simulink model "Control_discreto_Dom_tiempo"  (R2023b)
settings: Solver=VariableStepAuto  StartTime=0.0  StopTime=15  FixedStep=0.0001  MaxStep=1e-3  RelTol=1e-3
values from neighbouring files (symbols this model uses):
  ba = Jeq * n * wn    [PolosPID.m]
  id_consigna = 0.5    [RdLazoCorriente.m]
  ketita = double(sol.ketita_s)    [PIDPolosObsReducidoEst.m]    (also in PolosObsReducidoEst.m)
  kew = double(sol.kew_s)    [PIDPolosObsReducidoEst.m]    (also in PolosObsReducidoEst.m)
  kewint = double(sol.kewint_s)    [PIDPolosObsReducidoEst.m]    (also in PolosObsReducidoEst.m = 0)
  Ksa = Jeq * n * wn^2    [PolosPID.m]
  Ksia = Jeq * wn^3    [PolosPID.m]
  Ra_prima = Lq/Tau    [RaLazoControlCorriente.m]
  Rd_prima = Ld/Tau_d    [RdLazoCorriente.m]
  Ts = 0.0001    [TustinPID.m]
undefined symbols (not defined in the file or in its folder): alfa, beq, Cts, ee_sli_rtmsupport, g, gcbh, i0_consigna, id0, io0, iq0, Ismax, Isnom, Jeq, KEeq, kl, KTeq, lambda_m, Ld, Lls, Lq, Pp, r, R0_prima, Rs, Rts_amb, tita0, Tqnom, Ts0, Tsmax, Vflnom, Wlnom, wm0, Wmnom
libraries: SignalEditorBlockLib x3, dspsigops x1, spsabctoAlphaBetaZeroLib x1
settings Model: Creator=Julian  LastModifiedBy=Gustavo

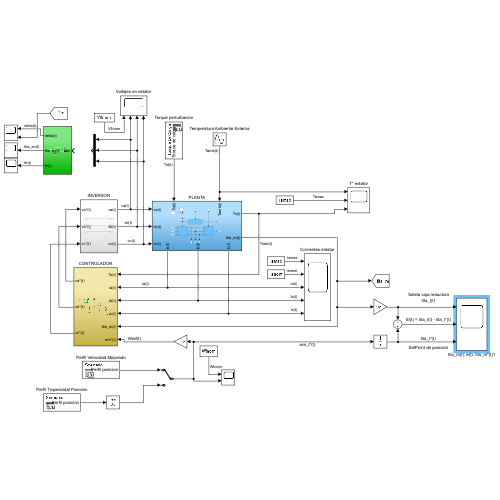
[thumbnail: Simulink's stored preview of the top-level diagram]
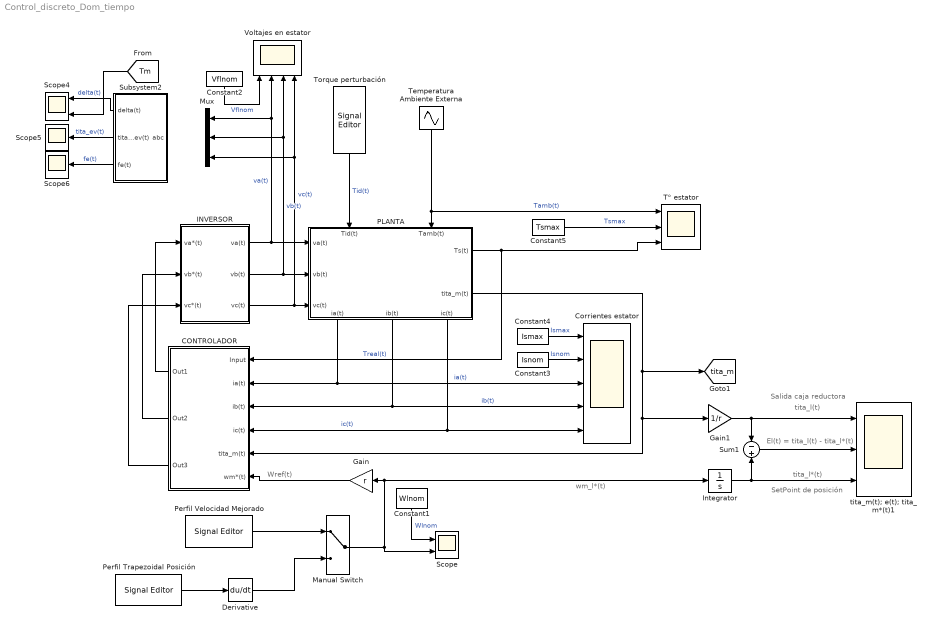
== system Control_discreto_Dom_tiempo ==
  note: SetPoint de posición
  note: Wref(t)
  note: Salida caja reductora
  note: El(t) = tita_l(t) - tita_l*(t)
  note: tita_l*(t)
  note: wm_l*(t)
  note: tita_l(t)
  CONTROLADOR : Subsystem
  Constant1 : Constant  Value=Wlnom
  Constant2 : Constant  Value=Vflnom
  Constant3 : Constant  Value=Isnom
  Constant4 : Constant  Value=Ismax
  Constant5 : Constant  Value=Tsmax
  Corrientes estator : Scope  NumInputPorts=5
  Derivative : Derivative
  Gain : Gain  Gain=r
  Gain1 : Gain  Gain=1/r
  INVERSOR : Subsystem
  Integrator : Integrator
  Manual Switch : ManualSwitch
  Mux : Mux  Inputs=3
  PLANTA : Subsystem
      settings: PortSchema="{\"entries\":[{\"content\":{\"sides\":[{\"content\":{\"connectorIds\":[\"In1\",\"In2\",\"In3\"]},\"type\":\"ConnectorPlacement.EquallySpacedRectSide\",\"uuid\":\"c9ff8e03-575d-49b6-9d53-263c6173ec7a\"},{\"content\":{\"connectorIds\":[\"Out1\",\"Out2\"],\"side\":\"RIGHT\"},\"type\":\"ConnectorPlacement.EquallySpacedRectSide\",\"uuid\":\"b812656a-111e-4032-91bd-eba1e3276cdf\"},{\"content\":{\"connectorIds\":[\"In4\",\"In5\"],\"side\":\"TOP\"},\"type\":\"ConnectorPlacement.EquallySpacedRectSide\",\"uuid\":\"1a03caaa-7f6e-4ad3-ab54-ee47607f786a\"},{\"content\":{\"connectorIds\":[\"Out3\",\"Out4\",\"Out5\"],\"side\":\"BOTTOM\"},\"type\":\"ConnectorPlacement.EquallySpacedRectSide\",\"uuid\":\"9d23a867-d392-4f38-a76b-2655c4618fc4\"}]},\"type\":\"ConnectorPlacement.EquallySpacedConnector\",\"uuid\":\"9323b1ce-1fa4-461e-b8aa-3e94b35b1dab\"}],\"packageUris\":[\"http://schema.mathworks.com/mf0/Connector/R2020b\"],\"version\":\"1.0\"}"
  Perfil Trapezoidal Posición : SignalEditorBlockLib/Signal Editor  FileName=Perfil trapezoidal de posicion.mat  ActiveScenario=Scenario  ActiveSignal=Perfil posicion  IsBus=off  OutputBusObjectStr=Bus: BusObject  SampleTime=0  ZeroCross=off  OutputAfterFinalValue=Setting to zero  Unit=inherit  PreserveSignalName=on  ApplySigPropsToAllScenarios=on  ApplySigPropsToAllSignals=off
  Perfil Velocidad Mejorado : SignalEditorBlockLib/Signal Editor  FileName=PerfilTrapezoidalVelocidadMejorado.mat  ActiveScenario=Scenario  ActiveSignal=Perfil posicion  IsBus=off  OutputBusObjectStr=Bus: BusObject  SampleTime=0  ZeroCross=off  OutputAfterFinalValue=Setting to zero  Unit=inherit  PreserveSignalName=on  ApplySigPropsToAllScenarios=on  ApplySigPropsToAllSignals=off
  Scope : Scope  NumInputPorts=2
  Scope4 : Scope  NumInputPorts=2
  Scope5 : Scope
  Scope6 : Scope
  Subsystem2 : Subsystem
  Sum1 : Sum  Inputs=-|+
  Temperatura Ambiente Externa : Sin  Bias=40  Frequency=2*pi/15  Phase=pi/2  SampleTime=0
  Torque perturbación : SignalEditorBlockLib/Signal Editor  FileName=Torque de carga Tdl(t).mat  ActiveScenario=TorqueDeCarga  ActiveSignal=Torque de carga  IsBus=off  OutputBusObjectStr=Bus: BusObject  SampleTime=0  ZeroCross=off  OutputAfterFinalValue=Setting to zero  Unit=N*m  PreserveSignalName=on  ApplySigPropsToAllScenarios=on  ApplySigPropsToAllSignals=off
  T° estator : Scope  NumInputPorts=3
  Voltajes en estator : Scope  NumInputPorts=4
  tita_m(t); e(t); tita_m*(t)1 : Scope  NumInputPorts=3
  tag scope: tita_m=global
  wires:
  INVERSOR/1(va(t)) -> PLANTA/1(va(t)), Voltajes en estator/2, Mux/1  "va(t)"
  INVERSOR/2(vb(t)) -> PLANTA/2(vb(t)), Mux/2, Voltajes en estator/3  "vb(t)"
  INVERSOR/3(vc(t)) -> Voltajes en estator/4, Mux/3, PLANTA/3(vc(t))  "vc(t)"
  CONTROLADOR/1(Out1) -> INVERSOR/1(va*(t))
  CONTROLADOR/2(Out2) -> INVERSOR/2(vb*(t))
  CONTROLADOR/3(Out3) -> INVERSOR/3(vc*(t))
  Gain/1 -> CONTROLADOR/6(wm*(t))
  PLANTA/2(tita_m(t)) -> CONTROLADOR/5(tita_m(t)), Gain1/1, [tita_m]
  Gain1/1 -> tita_m(t); e(t); tita_m*(t)1/1, Sum1/1
  Sum1/1 -> tita_m(t); e(t); tita_m*(t)1/2
  Integrator/1 -> Sum1/2, tita_m(t); e(t); tita_m*(t)1/3
  Temperatura Ambiente Externa/1 -> PLANTA/5(Tamb(t)), T° estator/1  "Tamb(t)"
  Torque perturbación/1 -> PLANTA/4(Tid(t))  "Tid(t)"
  PLANTA/5(ic(t)) -> Corrientes estator/5, CONTROLADOR/4(ic(t))  "ic(t)"
  PLANTA/4(ib(t)) -> Corrientes estator/4, CONTROLADOR/3(ib(t))  "ib(t)"
  PLANTA/3(ia(t)) -> Corrientes estator/3, CONTROLADOR/2(ia(t))  "ia(t)"
  Manual Switch/1 -> Integrator/1, Gain/1, Scope/2
  Perfil Trapezoidal Posición/1 -> Derivative/1
  Perfil Velocidad Mejorado/1 -> Manual Switch/1
  Constant1/1 -> Scope/1  "Wlnom"
  Constant2/1 -> Voltajes en estator/1  "Vflnom"
  Constant3/1 -> Corrientes estator/2  "Isnom"
  Constant4/1 -> Corrientes estator/1  "Ismax"
  Constant5/1 -> T° estator/2  "Tsmax"
  Derivative/1 -> Manual Switch/2
  PLANTA/1(Ts(t)) -> CONTROLADOR/1(Input), T° estator/3  "Treal(t)"
  Subsystem2/1(delta(t)) -> Scope4/1  "delta(t)"
  Subsystem2/2(tita_ev(t)) -> Scope5/1  "tita_ev(t)"
  Subsystem2/3(fe(t)) -> Scope6/1  "fe(t)"
  [Tm] -> Scope4/2

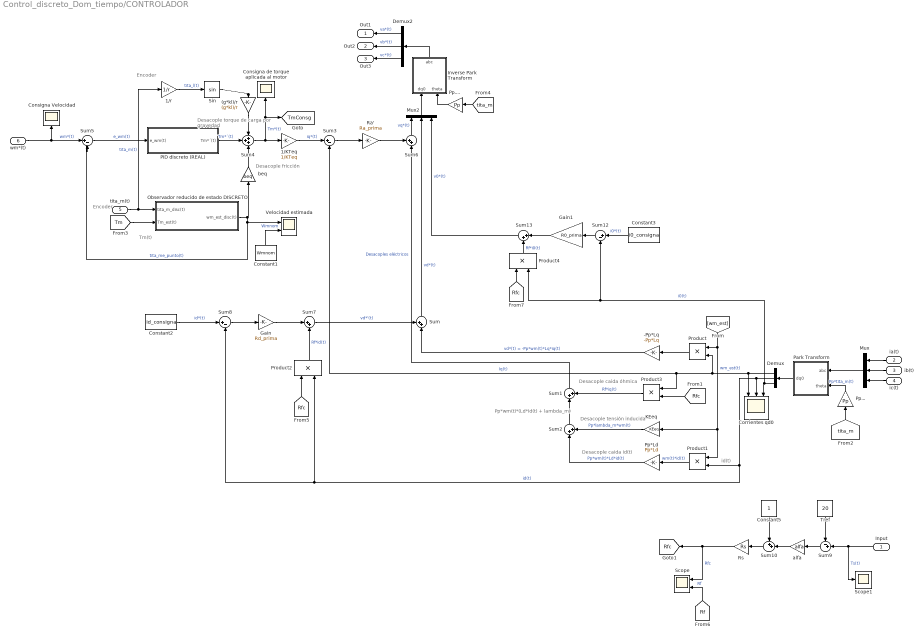
== system Control_discreto_Dom_tiempo/CONTROLADOR ==
  note: id(t)
  note: Desacople caida id(t)
  note: Encoder
  note: Desacople caida óhmica
  note: Desacople fricción
  note: Tm(t)
  note: Desacople tensión inducida
  note: Pp*wm(t)*(Ld*Id(t) + lambda_m)
  note: Encoder
  note: Desacople torque
      | de carga por gravedad
  Input : Inport
  ia(t) : Inport  Port=2
  ib(t) : Inport  Port=3
  ic(t) : Inport  Port=4
  tita_m(t) : Inport  Port=5
  wm*(t) : Inport  Port=6
  (g*kl)/r : Gain  Gain=(g*kl)/r
  -Pp*Lq : Gain  Gain=-Pp*Lq
  1/KTeq : Gain  Gain=1/KTeq
  1/r : Gain  Gain=1/r
  Consigna Velocidad : Scope
  Consigna de torque aplicada al motor : Scope
  Constant1 : Constant  Value=Wmnom
  Constant2 : Constant  Value=id_consigna
  Constant3 : Constant  Value=i0_consigna
  Constant5 : Constant
  Corrientes qd0 : Scope  NumInputPorts=3
  Demux : Demux  Outputs=3
  Demux2 : Demux  Outputs=3
  Gain : Gain  Gain=Rd_prima
  Gain1 : Gain  Gain=R0_prima
  Inverse Park Transform : Subsystem  AncestorBlock=|  LoadFcn=ee_sli_rtmsupport( 'loadfcn', gcbh );  mask(Inverse Park Transform){AxisAlignment=Q-axis, PowerInvariant=off}
      | ee_sl_lib/Mathematical
      | Transforms/Inverse
      | Park Transform
      mask prompts: AxisAlignment "physmod:ee:library:comments:control:eeTransforms:PhaseaAxisAlignment_MP"; PowerInvariant "physmod:ee:library:comments:control:eeTransforms:PowerInvariant_MP"
      mask help: physmod:ee:library:comments:control:eeTransforms:InverseParkTransform_MD
      mask init:
      | if PowerInvariant==0
      |     K1 = 1;
      |     K2 = 1;
      | else
      |     K1 = 1/sqrt(2);
      |     K2 = sqrt(2/3);
      | end
      | 
      | switch AxisAlignment
      |     case 'Q-axis'
      |         Offset = 0;
      |     case 'D-axis'
      |         Offset = pi/2;
      |     otherwise
      | end
      settings: CopyFcn=ee_sli_rtmsupport( 'copyfcn', gcbh );  DeleteFcn=ee_sli_rtmsupport( 'deletefcn', gcbh );  ModelCloseFcn=ee_sli_rtmsupport( 'modelclosefcn', gcbh );  PostSaveFcn=ee_sli_rtmsupport( 'postsavefcn', gcbh );  PreCopyFcn=ee_sli_rtmsupport( 'precopyfcn', gcbh );  OpenFcn=ee_sli_rtmsupport( 'openfcn', gcbh );  CloseFcn=ee_sli_rtmsupport( 'closefcn', gcbh );  PreDeleteFcn=ee_sli_rtmsupport( 'predeletefcn', gcbh );
      settings: LibrarySourceBlock=|
      | ee_sl_lib/Mathematical
      | Transforms/Inverse
      | Park Transform
      mask Help: web(nesl_help(gcbh))
      mask TypeOptions AxisAlignment: physmod:ee:library:comments:control:eeTransforms:Q0x2DAxis_PV | physmod:ee:library:comments:control:eeTransforms:D0x2DAxis_PV
      mask DialogControl AxisAlignment Prompt: Phase-a axis alignment
      mask DialogControl PowerInvariant Prompt: Power invariant
      mask Display: ee.mask.drawInverseParkTransform();
  KEeq : Gain  Gain=KEeq
  Mux : Mux  Inputs=3
  Mux2 : Mux  Inputs=3
  Observador reducido de estado DISCRETO : Subsystem
  PID discreto (REAL) : Subsystem
  Park Transform : Subsystem  AncestorBlock=ee_sl_lib/Mathematical Transforms/Park Transform  LoadFcn=ee_sli_rtmsupport( 'loadfcn', gcbh );  mask(Park Transform){AxisAlignment=Q-axis, PowerInvariant=off}
      mask prompts: AxisAlignment "physmod:ee:library:comments:control:eeTransforms:PhaseaAxisAlignment_MP"; PowerInvariant "physmod:ee:library:comments:control:eeTransforms:PowerInvariant_MP"
      mask help: physmod:ee:library:comments:control:eeTransforms:ParkTransform_MD
      mask init:
      | if PowerInvariant==0
      |     K1 = 0.5;
      |     K2 = 2/3;
      | else
      |     K1 = 1/sqrt(2);
      |     K2 = sqrt(2/3);
      | end
      | 
      | switch AxisAlignment
      |     case 'Q-axis'
      |         Offset = 0;
      |     case 'D-axis'
      |         Offset = pi/2;
      |     otherwise
      | end
      settings: CopyFcn=ee_sli_rtmsupport( 'copyfcn', gcbh );  DeleteFcn=ee_sli_rtmsupport( 'deletefcn', gcbh );  ModelCloseFcn=ee_sli_rtmsupport( 'modelclosefcn', gcbh );  PostSaveFcn=ee_sli_rtmsupport( 'postsavefcn', gcbh );  PreCopyFcn=ee_sli_rtmsupport( 'precopyfcn', gcbh );  OpenFcn=ee_sli_rtmsupport( 'openfcn', gcbh );  CloseFcn=ee_sli_rtmsupport( 'closefcn', gcbh );  PreDeleteFcn=ee_sli_rtmsupport( 'predeletefcn', gcbh );
      settings: LibrarySourceBlock=|
      | ee_sl_lib/Mathematical
      | Transforms/Park Transform
      mask Help: web(nesl_help(gcbh))
      mask TypeOptions AxisAlignment: physmod:ee:library:comments:control:eeTransforms:Q0x2DAxis_PV | physmod:ee:library:comments:control:eeTransforms:D0x2DAxis_PV
      mask DialogControl AxisAlignment Prompt: Phase-a axis alignment
      mask DialogControl PowerInvariant Prompt: Power invariant
      mask Display: ee.mask.drawParkTransform();
  Pp*Ld : Gain  Gain=Pp*Ld
  Pp... : Gain  Gain=Pp
  Pp.... : Gain  Gain=Pp
  Product{,1..4} (5 alike) : Product
  Ra' : Gain  Gain=Ra_prima
  Rs : Gain  Gain=Rs
  Scope : Scope  NumInputPorts=2
  Scope1 : Scope
  Sin : Trigonometry
  Sum : Sum  Inputs=++|
  Sum{1..2,7,13} (4 alike) : Sum  Inputs=|++
  Sum10 : Sum  Inputs=++|
  Sum{3,5,8,12} (4 alike) : Sum  Inputs=|+-
  Sum4 : Sum  Inputs=+++
  Sum6 : Sum  Inputs=++|
  Sum9 : Sum  Inputs=-+|
  Tref : Constant  Value=20
  Velocidad estimada : Scope  NumInputPorts=2
  alfa : Gain  Gain=alfa
  beq : Gain  Gain=beq
  Out1 : Outport
  Out2 : Outport  Port=2
  Out3 : Outport  Port=3
  tag scope: Rfc=global, TmConsg=global
  wires:
  Mux/1 -> Park Transform/1(abc)
  [tita_m] -> Pp..../1
  Pp..../1 -> Inverse Park Transform/2(theta)
  Demux2/2 -> Out2/1  "vb*(t)"
  Sum3/1 -> Ra'/1
  Demux2/1 -> Out1/1  "va*(t)"
  Product3/1 -> Sum1/2  "Rf*iq(t)"
  [tita_m] -> Pp.../1
  Ra'/1 -> Sum6/1
  Inverse Park Transform/1(abc) -> Demux2/1
  KEeq/1 -> Sum2/2  "Pp*lambda_m*wm(t)"
  Product1/1 -> Pp*Ld/1  "wm(t)*id(t)"
  Mux2/1 -> Inverse Park Transform/1(dq0)
  Sum2/1 -> Sum1/1
  wm*(t)/1 -> Sum5/1, Consigna Velocidad/1  "wm*(t)"
  Pp*Ld/1 -> Sum2/1  "Pp*wm(t)*Ld*id(t)"
  1/KTeq/1 -> Sum3/1  "iq*(t)"
  Product/1 -> -Pp*Lq/1
  ia(t)/1 -> Mux/1
  Park Transform/1(dq0) -> Demux/1
  Pp.../1 -> Park Transform/2(theta)  "Pp*tita_m(t)"
  Sum6/1 -> Mux2/1  "vq*(t)"
  Demux2/3 -> Out3/1  "vc*(t)"
  ib(t)/1 -> Mux/2
  tita_m(t)/1 -> Observador reducido de estado DISCRETO/1(tita_m_disc(t)), 1/r/1  "tita_m(t)"
  [Tm] -> Observador reducido de estado DISCRETO/2(Tm_est(t))
  ic(t)/1 -> Mux/3
  Sum5/1 -> PID discreto (REAL)/1(e_wm(t))  "e_wm(t)"
  Sum1/1 -> Sum6/2  "Desacoples eléctricos"
  PID discreto (REAL)/1(Tm*´(t)) -> Sum4/2  "Tm*´(t)"
  Sum4/1 -> 1/KTeq/1, Consigna de torque aplicada al motor/1, [TmConsg]  "Tm*(t)"
  beq/1 -> Sum4/3
  Observador reducido de estado DISCRETO/1(wm_est_disc(t)) -> Velocidad estimada/1, Sum5/2, beq/1  "tita_me_punto(t)"
  Demux/2 -> Product1/2, Sum8/2, Product2/2, Corrientes qd0/2  "id(t)"
  Demux/1 -> Product3/1, Sum3/2, Product/2, Corrientes qd0/1  "Iq(t)"
  1/r/1 -> Sin/1  "tita_l(t)"
  Sin/1 -> (g*kl)/r/1
  (g*kl)/r/1 -> Sum4/1
  [wm_est] -> Product/1, Product1/1, KEeq/1  "wm_est(t)"
  Constant1/1 -> Velocidad estimada/2  "Wmnom"
  Sum/1 -> Mux2/2  "vd*(t)"
  -Pp*Lq/1 -> Sum/2  "vd*(t) = -Pp*wm(t)*Lq*iq(t)"
  Product2/1 -> Sum7/2  "Rf*id(t)"
  Gain/1 -> Sum7/1
  Constant2/1 -> Sum8/1  "id*(t)"
  [Rfc] -> Product2/1
  [Rfc] -> Product3/2
  Tref/1 -> Sum9/1
  Rs/1 -> Scope/1, [Rfc]  "Rfc"
  alfa/1 -> Sum10/2
  Sum10/1 -> Rs/1
  Sum9/1 -> alfa/1
  Constant5/1 -> Sum10/1
  Input/1 -> Scope1/1, Sum9/2  "Ts(t)"
  [Rf] -> Scope/2  "Rf"
  Sum7/1 -> Sum/1  "vd*'(t)"
  Sum8/1 -> Gain/1
  Product4/1 -> Sum13/2  "Rf*i0(t)"
  Constant3/1 -> Sum12/1  "i0*(t)"
  Sum12/1 -> Gain1/1
  Demux/3 -> Product4/2, Sum12/2, Corrientes qd0/3  "i0(t)"
  Gain1/1 -> Sum13/1
  [Rfc] -> Product4/1
  Sum13/1 -> Mux2/3  "v0*(t)"

== system Control_discreto_Dom_tiempo/INVERSOR ==
  va*(t) : Inport
  vb*(t) : Inport  Port=2
  vc*(t) : Inport  Port=3
  va(t) : Outport
  vb(t) : Outport  Port=2
  vc(t) : Outport  Port=3
  wires:
  vc*(t)/1 -> vc(t)/1  "vc(t)"
  va*(t)/1 -> va(t)/1  "va(t)"
  vb*(t)/1 -> vb(t)/1  "vb(t)"

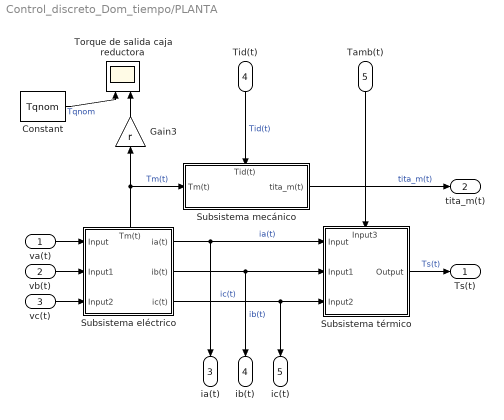
== system Control_discreto_Dom_tiempo/PLANTA ==
  va(t) : Inport
  vb(t) : Inport  Port=2
  vc(t) : Inport  Port=3
  Tid(t) : Inport  Port=4
  Tamb(t) : Inport  Port=5
  Constant : Constant  Value=Tqnom
  Gain3 : Gain  Gain=r
  Subsistema eléctrico : Subsystem
      settings: PortSchema="{\"entries\":[{\"content\":{\"sides\":[{\"content\":{\"connectorIds\":[\"In1\",\"In2\",\"In3\"]},\"type\":\"ConnectorPlacement.EquallySpacedRectSide\",\"uuid\":\"55314de5-b6ab-4161-b15d-819ac9b3d610\"},{\"content\":{\"connectorIds\":[\"Out1\",\"Out2\",\"Out3\"],\"side\":\"RIGHT\"},\"type\":\"ConnectorPlacement.EquallySpacedRectSide\",\"uuid\":\"6d89c228-26ff-4db5-b942-5bfef0be2fde\"},{\"content\":{\"connectorIds\":[\"Out4\"],\"side\":\"TOP\"},\"type\":\"ConnectorPlacement.EquallySpacedRectSide\",\"uuid\":\"a52f3ca3-a7f6-4886-b92b-9c9e6a107711\"}]},\"type\":\"ConnectorPlacement.EquallySpacedConnector\",\"uuid\":\"22991da4-d60d-4ddc-8bfe-b68e23663f11\"}],\"packageUris\":[\"http://schema.mathworks.com/mf0/Connector/R2020b\"],\"version\":\"1.0\"}"
  Subsistema mecánico : Subsystem
      settings: PortSchema="{\"entries\":[{\"content\":{\"sides\":[{\"content\":{\"connectorIds\":[\"In1\"]},\"type\":\"ConnectorPlacement.EquallySpacedRectSide\",\"uuid\":\"db0c31ff-fb9a-4cce-bd75-6b297d65744d\"},{\"content\":{\"connectorIds\":[\"Out1\"],\"side\":\"RIGHT\"},\"type\":\"ConnectorPlacement.EquallySpacedRectSide\",\"uuid\":\"ab44173d-bb84-4ea2-b7b7-ef15b1ff9d5e\"},{\"content\":{\"connectorIds\":[\"In2\"],\"side\":\"TOP\"},\"type\":\"ConnectorPlacement.EquallySpacedRectSide\",\"uuid\":\"a2ba5669-abba-4e87-b14b-37ec0d904023\"}]},\"type\":\"ConnectorPlacement.EquallySpacedConnector\",\"uuid\":\"7722c9ef-afaa-4930-9e2a-97c0dfb446ab\"}],\"packageUris\":[\"http://schema.mathworks.com/mf0/Connector/R2020b\"],\"version\":\"1.0\"}"
  Subsistema térmico : Subsystem
      settings: PortSchema="{\"entries\":[{\"content\":{\"sides\":[{\"content\":{\"connectorIds\":[\"In1\",\"In2\",\"In3\"]},\"type\":\"ConnectorPlacement.EquallySpacedRectSide\",\"uuid\":\"499bb5e3-da94-498d-be5e-1974ba0b4a58\"},{\"content\":{\"connectorIds\":[\"Out1\"],\"side\":\"RIGHT\"},\"type\":\"ConnectorPlacement.EquallySpacedRectSide\",\"uuid\":\"13ea5dea-e51e-4770-b579-88e3e6e50884\"},{\"content\":{\"connectorIds\":[\"In4\"],\"side\":\"TOP\"},\"type\":\"ConnectorPlacement.EquallySpacedRectSide\",\"uuid\":\"72517ed1-a98f-428e-86e2-c370e237c602\"}]},\"type\":\"ConnectorPlacement.EquallySpacedConnector\",\"uuid\":\"7e0eda24-12d6-49d0-ad1f-024c88e78140\"}],\"packageUris\":[\"http://schema.mathworks.com/mf0/Connector/R2020b\"],\"version\":\"1.0\"}"
  Torque de salida caja reductora : Scope  NumInputPorts=2
  Ts(t) : Outport
  tita_m(t) : Outport  Port=2
  ia(t) : Outport  Port=3
  ib(t) : Outport  Port=4
  ic(t) : Outport  Port=5
  wires:
  Tamb(t)/1 -> Subsistema térmico/4(Input3)
  Subsistema eléctrico/3(ic(t)) -> Subsistema térmico/3(Input2), ic(t)/1  "ic(t)"
  Subsistema eléctrico/1(ia(t)) -> Subsistema térmico/1(Input), ia(t)/1  "ia(t)"
  Subsistema térmico/1(Output) -> Ts(t)/1  "Ts(t)"
  Subsistema eléctrico/4(Tm(t)) -> Gain3/1, Subsistema mecánico/1(Tm(t))  "Tm(t)"
  Subsistema eléctrico/2(ib(t)) -> Subsistema térmico/2(Input1), ib(t)/1  "ib(t)"
  Subsistema mecánico/1(tita_m(t)) -> tita_m(t)/1  "tita_m(t)"
  va(t)/1 -> Subsistema eléctrico/1(Input)
  vb(t)/1 -> Subsistema eléctrico/2(Input1)
  Tid(t)/1 -> Subsistema mecánico/2(Tid(t))  "Tid(t)"
  vc(t)/1 -> Subsistema eléctrico/3(Input2)
  Gain3/1 -> Torque de salida caja reductora/2
  Constant/1 -> Torque de salida caja reductora/1  "Tqnom"

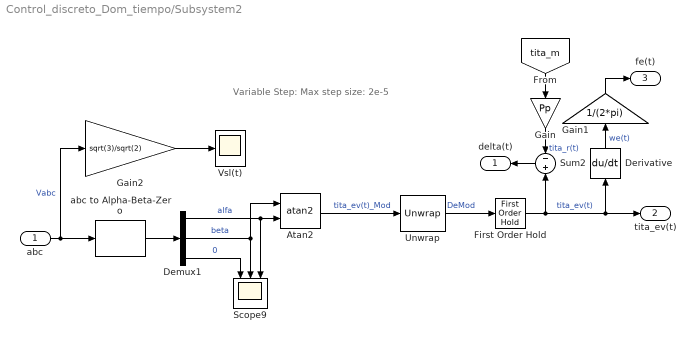
== system Control_discreto_Dom_tiempo/Subsystem2 ==
  note: Variable Step: Max step size: 2e-5
  abc : Inport
  Atan2 : Trigonometry  Operator=atan2
  Demux1 : Demux  Outputs=3
  Derivative : Derivative
  First Order Hold : FirstOrderHold  ErrorTolerance=inf  AllowContinuousInput=on
  Gain : Gain  Gain=Pp
  Gain1 : Gain  Gain=1/(2*pi)
  Gain2 : Gain  Gain=sqrt(3)/sqrt(2)
  Scope9 : Scope  NumInputPorts=3
  Sum2 : Sum  Inputs=-|+
  Unwrap : dspsigops/Unwrap  tol=1.2*pi  InputProcessing=Columns as channels (frame based)  running=off
  Vsl(t) : Scope
  abc to Alpha-Beta-Zero : spsabctoAlphaBetaZeroLib/abc to Alpha-Beta-Zero
  delta(t) : Outport
  tita_ev(t) : Outport  Port=2
  fe(t) : Outport  Port=3
  wires:
  Demux1/1 -> Scope9/3, Atan2/2  "alfa"
  abc to Alpha-Beta-Zero/1 -> Demux1/1
  Atan2/1 -> Unwrap/1  "tita_ev(t)_Mod"
  Demux1/2 -> Scope9/2, Atan2/1  "beta"
  abc/1 -> Gain2/1, abc to Alpha-Beta-Zero/1  "Vabc"
  Demux1/3 -> Scope9/1  "0"
  Derivative/1 -> Gain1/1  "we(t)"
  Gain1/1 -> fe(t)/1
  [tita_m] -> Gain/1
  Gain/1 -> Sum2/1  "tita_r(t)"
  Sum2/1 -> delta(t)/1
  Unwrap/1 -> First Order Hold/1  "DeMod"
  First Order Hold/1 -> tita_ev(t)/1, Derivative/1, Sum2/2  "tita_ev(t)"
  Gain2/1 -> Vsl(t)/1

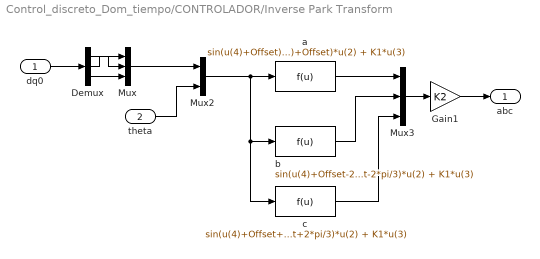
== system Control_discreto_Dom_tiempo/CONTROLADOR/Inverse Park Transform ==
  dq0 : Inport
  theta : Inport  Port=2
  Demux : Demux  Outputs=3
  Gain1 : Gain  Gain=K2
  Mux : Mux  Inputs=3
  Mux2 : Mux  Inputs=2
  Mux3 : Mux  Inputs=3
  a : Fcn  Expr=sin(u(4)+Offset)*u(1) + cos(u(4)+Offset)*u(2) + K1*u(3)
  b : Fcn  Expr=sin(u(4)+Offset-2*pi/3)*u(1) + cos(u(4)+Offset-2*pi/3)*u(2) + K1*u(3)
  c : Fcn  Expr=sin(u(4)+Offset+2*pi/3)*u(1) + cos(u(4)+Offset+2*pi/3)*u(2) + K1*u(3)
  abc : Outport  VectorParamsAs1DForOutWhenUnconnected=off
  wires:
  a/1 -> Mux3/1
  Mux3/1 -> Gain1/1
  Mux2/1 -> a/1, c/1, b/1
  theta/1 -> Mux2/2
  c/1 -> Mux3/3
  Gain1/1 -> abc/1
  b/1 -> Mux3/2
  dq0/1 -> Demux/1
  Demux/1 -> Mux/2
  Demux/2 -> Mux/1
  Demux/3 -> Mux/3
  Mux/1 -> Mux2/1

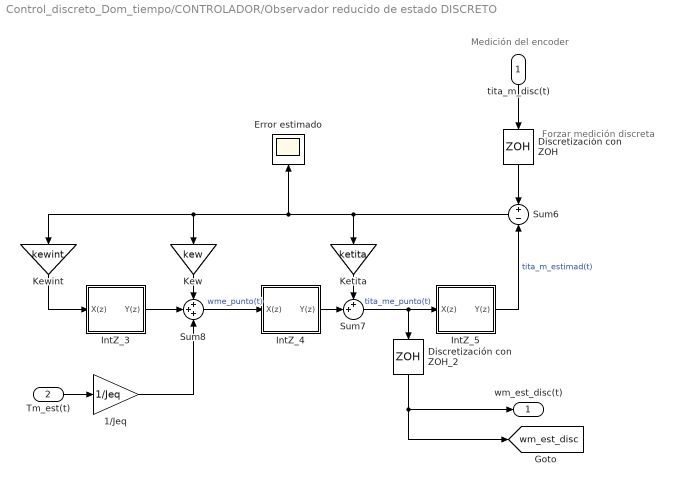
== system Control_discreto_Dom_tiempo/CONTROLADOR/Observador reducido de estado DISCRETO ==
  note: Forzar medición discreta
  note: Medición del encoder
  tita_m_disc(t) : Inport
  Tm_est(t) : Inport  Port=2
  1/Jeq : Gain  Gain=1/Jeq
  Discretización con ZOH : ZeroOrderHold  SampleTime=Ts
  Discretización con ZOH_2 : ZeroOrderHold  SampleTime=Ts
  Error estimado : Scope
  IntZ_3 : Subsystem
  IntZ_4 : Subsystem
  IntZ_5 : Subsystem
  Ketita : Gain  Gain=ketita
  Kew : Gain  Gain=kew
  Kewint : Gain  Gain=kewint
  Sum6 : Sum  Inputs=+-
  Sum7 : Sum  Inputs=++|
  Sum8 : Sum  Inputs=+++
  wm_est_disc(t) : Outport
  tag scope: wm_est_disc=global
  wires:
  Sum7/1 -> IntZ_5/1(X(z)), Discretización con ZOH_2/1  "tita_me_punto(t)"
  Sum6/1 -> Kewint/1, Kew/1, Error estimado/1, Ketita/1
  IntZ_5/1(Y(z)) -> Sum6/2  "tita_m_estimad(t)"
  Kew/1 -> Sum8/1
  Ketita/1 -> Sum7/1
  Sum8/1 -> IntZ_4/1(X(z))  "wme_punto(t)"
  tita_m_disc(t)/1 -> Discretización con ZOH/1
  1/Jeq/1 -> Sum8/3
  IntZ_4/1(Y(z)) -> Sum7/2
  IntZ_3/1(Y(z)) -> Sum8/2
  Kewint/1 -> IntZ_3/1(X(z))
  Discretización con ZOH/1 -> Sum6/1
  Tm_est(t)/1 -> 1/Jeq/1
  Discretización con ZOH_2/1 -> [wm_est_disc], wm_est_disc(t)/1

== system Control_discreto_Dom_tiempo/CONTROLADOR/PID discreto (REAL) ==
  note: P
  note: D
  note: I
  e_wm(t) : Inport
  Discretización con ZOH : ZeroOrderHold  SampleTime=Ts
  Discretización con ZOH1 : ZeroOrderHold  SampleTime=Ts
  IntZ_1 : Subsystem
  Ksa : Gain  Gain=Ksa
  Ksia : Gain  Gain=Ksia
  Sum4 : Sum  Inputs=+++
  ba : Gain  Gain=ba
  intZ_2 : Subsystem
  Tm*´(t) : Outport
  wires:
  Ksia/1 -> Sum4/1
  IntZ_1/1(Y(z)) -> intZ_2/1(X(z)), Ksa/1  "e_titam(t)"
  e_wm(t)/1 -> Discretización con ZOH/1
  intZ_2/1(Y(z)) -> Ksia/1
  Ksa/1 -> Sum4/2
  ba/1 -> Sum4/3
  Sum4/1 -> Discretización con ZOH1/1  "Tm*´(t)"
  Discretización con ZOH/1 -> IntZ_1/1(X(z)), ba/1
  Discretización con ZOH1/1 -> Tm*´(t)/1

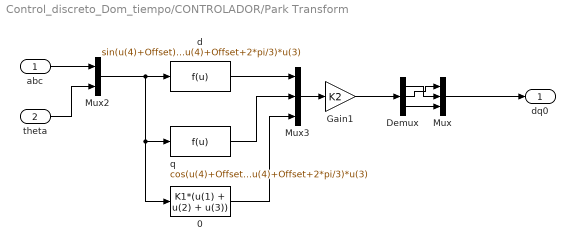
== system Control_discreto_Dom_tiempo/CONTROLADOR/Park Transform ==
  abc : Inport
  theta : Inport  Port=2
  0 : Fcn  Expr=K1*(u(1) + u(2) + u(3))
  Demux : Demux  Outputs=3
  Gain1 : Gain  Gain=K2
  Mux : Mux  Inputs=3
  Mux2 : Mux  Inputs=2
  Mux3 : Mux  Inputs=3
  d : Fcn  Expr=sin(u(4)+Offset)*u(1) + sin(u(4)+Offset-2*pi/3)*u(2) + sin(u(4)+Offset+2*pi/3)*u(3)
  q : Fcn  Expr=cos(u(4)+Offset)*u(1) + cos(u(4)+Offset-2*pi/3)*u(2) + cos(u(4)+Offset+2*pi/3)*u(3)
  dq0 : Outport  VectorParamsAs1DForOutWhenUnconnected=off
  wires:
  0/1 -> Mux3/3
  Mux3/1 -> Gain1/1
  Mux2/1 -> 0/1, q/1, d/1
  theta/1 -> Mux2/2
  q/1 -> Mux3/2
  d/1 -> Mux3/1
  abc/1 -> Mux2/1
  Demux/3 -> Mux/3
  Demux/1 -> Mux/2
  Demux/2 -> Mux/1
  Mux/1 -> dq0/1
  Gain1/1 -> Demux/1

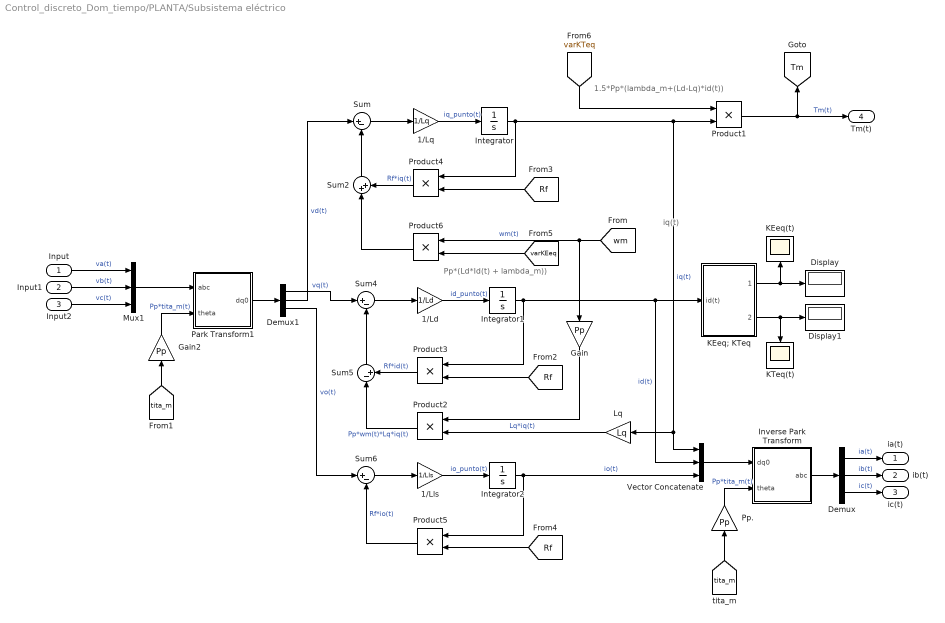
== system Control_discreto_Dom_tiempo/PLANTA/Subsistema eléctrico ==
  note: 1.5*Pp*(lambda_m+(Ld-Lq)*id(t))
  note: iq(t)
  note: Pp*(Ld*Id(t) + lambda_m))
  Input : Inport
  Input1 : Inport  Port=2
  Input2 : Inport  Port=3
  1/Ld : Gain  Gain=1/Ld
  1/Lls : Gain  Gain=1/Lls
  1/Lq : Gain  Gain=1/Lq
  Demux : Demux  Outputs=3
  Demux1 : Demux  Outputs=3
  Display : Display
  Display1 : Display
  Gain : Gain  Gain=Pp
  Gain2 : Gain  Gain=Pp
  Integrator : Integrator  InitialCondition=iq0
  Integrator1 : Integrator  InitialCondition=id0
  Integrator2 : Integrator  InitialCondition=io0
  Inverse Park Transform : Subsystem  AncestorBlock=|  LoadFcn=ee_sli_rtmsupport( 'loadfcn', gcbh );  mask(Inverse Park Transform){AxisAlignment=Q-axis, PowerInvariant=off}
      | ee_sl_lib/Mathematical
      | Transforms/Inverse
      | Park Transform
      mask prompts: AxisAlignment "physmod:ee:library:comments:control:eeTransforms:PhaseaAxisAlignment_MP"; PowerInvariant "physmod:ee:library:comments:control:eeTransforms:PowerInvariant_MP"
      mask help: physmod:ee:library:comments:control:eeTransforms:InverseParkTransform_MD
      mask init: same as Control_discreto_Dom_tiempo/CONTROLADOR/Inverse Park Transform
      settings: CopyFcn=ee_sli_rtmsupport( 'copyfcn', gcbh );  DeleteFcn=ee_sli_rtmsupport( 'deletefcn', gcbh );  ModelCloseFcn=ee_sli_rtmsupport( 'modelclosefcn', gcbh );  PostSaveFcn=ee_sli_rtmsupport( 'postsavefcn', gcbh );  PreCopyFcn=ee_sli_rtmsupport( 'precopyfcn', gcbh );  OpenFcn=ee_sli_rtmsupport( 'openfcn', gcbh );  CloseFcn=ee_sli_rtmsupport( 'closefcn', gcbh );  PreDeleteFcn=ee_sli_rtmsupport( 'predeletefcn', gcbh );
      settings: LibrarySourceBlock=|
      | ee_sl_lib/Mathematical
      | Transforms/Inverse
      | Park Transform
      mask Help: web(nesl_help(gcbh))
      mask TypeOptions AxisAlignment: physmod:ee:library:comments:control:eeTransforms:Q0x2DAxis_PV | physmod:ee:library:comments:control:eeTransforms:D0x2DAxis_PV
      mask DialogControl AxisAlignment Prompt: Phase-a axis alignment
      mask DialogControl PowerInvariant Prompt: Power invariant
      mask Display: ee.mask.drawInverseParkTransform();
  KEeq(t) : Scope
  KEeq; KTeq : Subsystem
  KTeq(t) : Scope
  Lq : Gain  Gain=Lq
  Mux1 : Mux  Inputs=3
  Park Transform1 : Subsystem  AncestorBlock=ee_sl_lib/Mathematical Transforms/Park Transform  LoadFcn=ee_sli_rtmsupport( 'loadfcn', gcbh );  mask(Park Transform){AxisAlignment=Q-axis, PowerInvariant=off}
      mask prompts: AxisAlignment "physmod:ee:library:comments:control:eeTransforms:PhaseaAxisAlignment_MP"; PowerInvariant "physmod:ee:library:comments:control:eeTransforms:PowerInvariant_MP"
      mask help: physmod:ee:library:comments:control:eeTransforms:ParkTransform_MD
      mask init: same as Control_discreto_Dom_tiempo/CONTROLADOR/Park Transform
      settings: CopyFcn=ee_sli_rtmsupport( 'copyfcn', gcbh );  DeleteFcn=ee_sli_rtmsupport( 'deletefcn', gcbh );  ModelCloseFcn=ee_sli_rtmsupport( 'modelclosefcn', gcbh );  PostSaveFcn=ee_sli_rtmsupport( 'postsavefcn', gcbh );  PreCopyFcn=ee_sli_rtmsupport( 'precopyfcn', gcbh );  OpenFcn=ee_sli_rtmsupport( 'openfcn', gcbh );  CloseFcn=ee_sli_rtmsupport( 'closefcn', gcbh );  PreDeleteFcn=ee_sli_rtmsupport( 'predeletefcn', gcbh );
      settings: LibrarySourceBlock=|
      | ee_sl_lib/Mathematical
      | Transforms/Park Transform
      mask Help: web(nesl_help(gcbh))
      mask TypeOptions AxisAlignment: physmod:ee:library:comments:control:eeTransforms:Q0x2DAxis_PV | physmod:ee:library:comments:control:eeTransforms:D0x2DAxis_PV
      mask DialogControl AxisAlignment Prompt: Phase-a axis alignment
      mask DialogControl PowerInvariant Prompt: Power invariant
      mask Display: ee.mask.drawParkTransform();
  Pp. : Gain  Gain=Pp
  Product{1..6} (6 alike) : Product
  Sum : Sum  Inputs=|+-
  Sum2 : Sum  Inputs=|++
  Sum4 : Sum  Inputs=|+-
  Sum5 : Sum  Inputs=|-+
  Sum6 : Sum  Inputs=|+-
  Vector Concatenate : Concatenate  NumInputs=3
  ia(t) : Outport
  ib(t) : Outport  Port=2
  ic(t) : Outport  Port=3
  Tm(t) : Outport  Port=4
  tag scope: Tm=global
  wires:
  Sum4/1 -> 1/Ld/1
  Demux1/1 -> Sum4/1  "vq(t)"
  Integrator/1 -> Product4/1, Product1/2, Lq/1, Vector Concatenate/1  "iq(t)"
  Product4/1 -> Sum2/2  "Rf*iq(t)"
  Pp./1 -> Inverse Park Transform/2(theta)  "Pp*tita_m(t)"
  Lq/1 -> Product2/2  "Lq*iq(t)"
  Sum/1 -> 1/Lq/1
  Sum2/1 -> Sum/2
  Demux1/3 -> Sum6/1  "vo(t)"
  Vector Concatenate/1 -> Inverse Park Transform/1(dq0)
  1/Ld/1 -> Integrator1/1  "id_punto(t)"
  Inverse Park Transform/1(abc) -> Demux/1
  1/Lls/1 -> Integrator2/1  "io_punto(t)"
  Sum5/1 -> Sum4/2
  Demux/3 -> ic(t)/1  "ic(t)"
  Demux/1 -> ia(t)/1  "ia(t)"
  Product3/1 -> Sum5/2  "Rf*id(t)"
  Demux/2 -> ib(t)/1  "ib(t)"
  Integrator2/1 -> Product5/1, Vector Concatenate/3  "io(t)"
  [tita_m] -> Pp./1
  Demux1/2 -> Sum/1  "vd(t)"
  Product6/1 -> Sum2/1
  Product5/1 -> Sum6/2  "Rf*io(t)"
  Product2/1 -> Sum5/1  "Pp*wm(t)*Lq*iq(t)"
  1/Lq/1 -> Integrator/1  "iq_punto(t)"
  Sum6/1 -> 1/Lls/1
  [wm] -> Product6/1, Gain/1  "wm(t)"
  Product1/1 -> Tm(t)/1, [Tm]  "Tm(t)"
  Input1/1 -> Mux1/2  "vb(t)"
  Gain2/1 -> Park Transform1/2(theta)  "Pp*tita_m(t)"
  Input2/1 -> Mux1/3  "vc(t)"
  Mux1/1 -> Park Transform1/1(abc)
  Input/1 -> Mux1/1  "va(t)"
  [tita_m] -> Gain2/1
  Park Transform1/1(dq0) -> Demux1/1
  [Rf] -> Product3/2
  [Rf] -> Product4/2
  [Rf] -> Product5/2
  Integrator1/1 -> Product3/1, KEeq; KTeq/1(id(t)), Vector Concatenate/2  "id(t)"
  KEeq; KTeq/2(KTeq(t)) -> Display1/1, KTeq(t)/1
  KEeq; KTeq/1(KEeq(t)) -> KEeq(t)/1, Display/1
  [varKEeq] -> Product6/2
  Gain/1 -> Product2/1
  [varKTeq] -> Product1/1

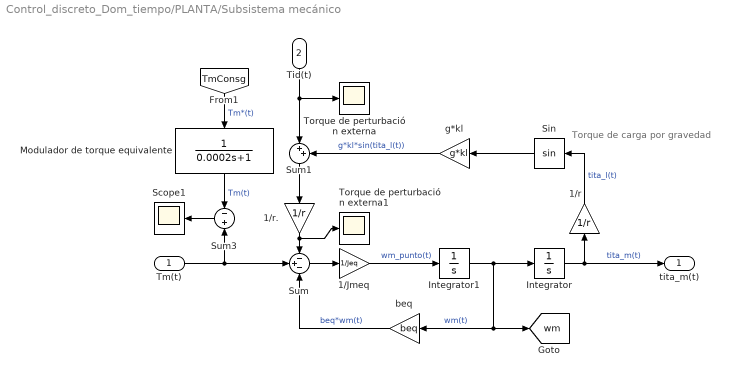
== system Control_discreto_Dom_tiempo/PLANTA/Subsistema mecánico ==
  note: Torque de carga por gravedad
  Tm(t) : Inport
  Tid(t) : Inport  Port=2
  1/Jmeq : Gain  Gain=1/Jeq
  1/r : Gain  Gain=1/r
  1/r. : Gain  Gain=1/r
  Integrator : Integrator  InitialCondition=tita0
  Integrator1 : Integrator  InitialCondition=wm0
  Modulador de torque equivalente : TransferFcn  Denominator=[0.0002 1]
  Scope1 : Scope
  Sin : Trigonometry
  Sum : Sum  Inputs=-+-
  Sum1 : Sum  Inputs=|++
  Sum3 : Sum  Inputs=-|+
  Torque de perturbación externa : Scope
  Torque de perturbación externa1 : Scope
  beq : Gain  Gain=beq
  g*kl : Gain  Gain=g*kl
  tita_m(t) : Outport
  tag scope: wm=global
  wires:
  Integrator/1 -> tita_m(t)/1, 1/r/1  "tita_m(t)"
  1/r./1 -> Torque de perturbación externa1/1, Sum/1
  Integrator1/1 -> beq/1, [wm], Integrator/1  "wm(t)"
  1/r/1 -> Sin/1  "tita_l(t)"
  Sin/1 -> g*kl/1
  Sum/1 -> 1/Jmeq/1
  1/Jmeq/1 -> Integrator1/1  "wm_punto(t)"
  beq/1 -> Sum/3  "beq*wm(t)"
  Tid(t)/1 -> Sum1/1, Torque de perturbación externa/1
  Sum1/1 -> 1/r./1
  g*kl/1 -> Sum1/2  "g*kl*sin(tita_l(t))"
  [TmConsg] -> Modulador de torque equivalente/1  "Tm*(t)"
  Sum3/1 -> Scope1/1
  Modulador de torque equivalente/1 -> Sum3/1  "Tm(t)"
  Tm(t)/1 -> Sum/2, Sum3/2

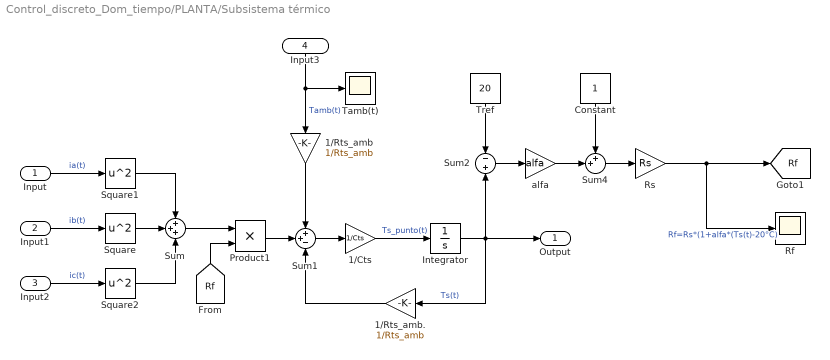
== system Control_discreto_Dom_tiempo/PLANTA/Subsistema térmico ==
  Input : Inport
  Input1 : Inport  Port=2
  Input2 : Inport  Port=3
  Input3 : Inport  Port=4
  1/Cts : Gain  Gain=1/Cts
  1/Rts_amb : Gain  Gain=1/Rts_amb
  1/Rts_amb. : Gain  Gain=1/Rts_amb
  Constant : Constant
  Integrator : Integrator  InitialCondition=Ts0
  Product1 : Product
  Rf : Scope
  Rs : Gain  Gain=Rs
  Square : Math  Operator=square
  Square1 : Math  Operator=square
  Square2 : Math  Operator=square
  Sum : Sum  Inputs=+++
  Sum1 : Sum  Inputs=++-
  Sum2 : Sum  Inputs=-+
  Sum4 : Sum  Inputs=++|
  Tamb(t) : Scope
  Tref : Constant  Value=20
  alfa : Gain  Gain=alfa
  Output : Outport
  tag scope: Rf=global
  wires:
  1/Rts_amb/1 -> Sum1/1
  Sum1/1 -> 1/Cts/1
  Product1/1 -> Sum1/2
  Sum/1 -> Product1/1
  Integrator/1 -> Sum2/2, Output/1, 1/Rts_amb./1  "Ts(t)"
  1/Cts/1 -> Integrator/1  "Ts_punto(t)"
  1/Rts_amb./1 -> Sum1/3
  Square/1 -> Sum/2
  Square1/1 -> Sum/1
  Square2/1 -> Sum/3
  Input/1 -> Square1/1  "ia(t)"
  Input1/1 -> Square/1  "ib(t)"
  Input2/1 -> Square2/1  "ic(t)"
  Sum2/1 -> alfa/1
  Constant/1 -> Sum4/1
  alfa/1 -> Sum4/2
  Rs/1 -> Rf/1, [Rf]  "Rf=Rs*(1+alfa*(Ts(t)-20°C)"
  [Rf] -> Product1/2
  Tref/1 -> Sum2/1
  Sum4/1 -> Rs/1
  Input3/1 -> 1/Rts_amb/1, Tamb(t)/1  "Tamb(t)"

== system Control_discreto_Dom_tiempo/CONTROLADOR/Observador reducido de estado DISCRETO/IntZ_3 ==
  note: H(z) = Y(z) / X(z) = (Ts/2) * (1+z^-1) / (1+z^-1)
  X(z) : Inport
  Gain : Gain  Gain=Ts/2
  Sum : Sum  Inputs=|++
  Sum1 : Sum  Inputs=|++
  Unit Delay : UnitDelay  SampleTime=-1  HasFrameUpgradeWarning=on
  Unit Delay1 : UnitDelay  SampleTime=-1  HasFrameUpgradeWarning=on
  Y(z) : Outport
  wires:
  Sum/1 -> Gain/1
  Sum1/1 -> Y(z)/1, Unit Delay1/1
  Gain/1 -> Sum1/1
  Unit Delay/1 -> Sum/2
  X(z)/1 -> Sum/1, Unit Delay/1
  Unit Delay1/1 -> Sum1/2

== system Control_discreto_Dom_tiempo/CONTROLADOR/Observador reducido de estado DISCRETO/IntZ_4 ==
  note: H(z) = Y(z) / X(z) = (Ts/2) * (1+z^-1) / (1+z^-1)
  X(z) : Inport
  Gain : Gain  Gain=Ts/2
  Sum : Sum  Inputs=|++
  Sum1 : Sum  Inputs=|++
  Unit Delay : UnitDelay  SampleTime=-1  HasFrameUpgradeWarning=on
  Unit Delay1 : UnitDelay  SampleTime=-1  HasFrameUpgradeWarning=on
  Y(z) : Outport
  wires:
  Unit Delay1/1 -> Sum1/2
  X(z)/1 -> Unit Delay/1, Sum/1
  Unit Delay/1 -> Sum/2
  Gain/1 -> Sum1/1
  Sum1/1 -> Unit Delay1/1, Y(z)/1
  Sum/1 -> Gain/1

== system Control_discreto_Dom_tiempo/CONTROLADOR/Observador reducido de estado DISCRETO/IntZ_5 ==
  note: H(z) = Y(z) / X(z) = (Ts/2) * (1+z^-1) / (1+z^-1)
  X(z) : Inport
  Gain : Gain  Gain=Ts/2
  Sum : Sum  Inputs=|++
  Sum1 : Sum  Inputs=|++
  Unit Delay : UnitDelay  SampleTime=-1  HasFrameUpgradeWarning=on
  Unit Delay1 : UnitDelay  SampleTime=-1  HasFrameUpgradeWarning=on
  Y(z) : Outport
  wires:
  Sum/1 -> Gain/1
  Sum1/1 -> Y(z)/1, Unit Delay1/1
  Gain/1 -> Sum1/1
  Unit Delay/1 -> Sum/2
  X(z)/1 -> Sum/1, Unit Delay/1
  Unit Delay1/1 -> Sum1/2

== system Control_discreto_Dom_tiempo/CONTROLADOR/PID discreto (REAL)/IntZ_1 ==
  note: H(z) = Y(z) / X(z) = (Ts/2) * (1+z^-1) / (1+z^-1)
  X(z) : Inport
  Gain : Gain  Gain=Ts/2
  Sum : Sum  Inputs=|++
  Sum1 : Sum  Inputs=|++
  Unit Delay : UnitDelay  SampleTime=-1  HasFrameUpgradeWarning=on
  Unit Delay1 : UnitDelay  SampleTime=-1  HasFrameUpgradeWarning=on
  Y(z) : Outport
  wires:
  Unit Delay1/1 -> Sum1/2
  X(z)/1 -> Unit Delay/1, Sum/1
  Unit Delay/1 -> Sum/2
  Gain/1 -> Sum1/1
  Sum1/1 -> Unit Delay1/1, Y(z)/1
  Sum/1 -> Gain/1

== system Control_discreto_Dom_tiempo/CONTROLADOR/PID discreto (REAL)/intZ_2 ==
  note: H(z) = Y(z) / X(z) = (Ts/2) * (1+z^-1) / (1+z^-1)
  X(z) : Inport
  Gain : Gain  Gain=Ts/2
  Sum : Sum  Inputs=|++
  Sum1 : Sum  Inputs=|++
  Unit Delay : UnitDelay  SampleTime=-1  HasFrameUpgradeWarning=on
  Unit Delay1 : UnitDelay  SampleTime=-1  HasFrameUpgradeWarning=on
  Y(z) : Outport
  wires:
  Sum/1 -> Gain/1
  Sum1/1 -> Y(z)/1, Unit Delay1/1
  Gain/1 -> Sum1/1
  Unit Delay/1 -> Sum/2
  X(z)/1 -> Sum/1, Unit Delay/1
  Unit Delay1/1 -> Sum1/2

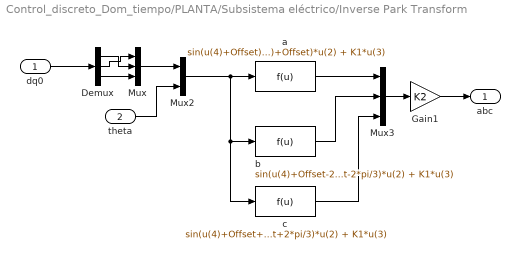
== system Control_discreto_Dom_tiempo/PLANTA/Subsistema eléctrico/Inverse Park Transform ==
  dq0 : Inport
  theta : Inport  Port=2
  Demux : Demux  Outputs=3
  Gain1 : Gain  Gain=K2
  Mux : Mux  Inputs=3
  Mux2 : Mux  Inputs=2
  Mux3 : Mux  Inputs=3
  a : Fcn  Expr=sin(u(4)+Offset)*u(1) + cos(u(4)+Offset)*u(2) + K1*u(3)
  b : Fcn  Expr=sin(u(4)+Offset-2*pi/3)*u(1) + cos(u(4)+Offset-2*pi/3)*u(2) + K1*u(3)
  c : Fcn  Expr=sin(u(4)+Offset+2*pi/3)*u(1) + cos(u(4)+Offset+2*pi/3)*u(2) + K1*u(3)
  abc : Outport  VectorParamsAs1DForOutWhenUnconnected=off
  wires:
  a/1 -> Mux3/1
  Mux3/1 -> Gain1/1
  Mux2/1 -> a/1, c/1, b/1
  theta/1 -> Mux2/2
  c/1 -> Mux3/3
  Gain1/1 -> abc/1
  b/1 -> Mux3/2
  Demux/2 -> Mux/1
  Demux/1 -> Mux/2
  Demux/3 -> Mux/3
  dq0/1 -> Demux/1
  Mux/1 -> Mux2/1

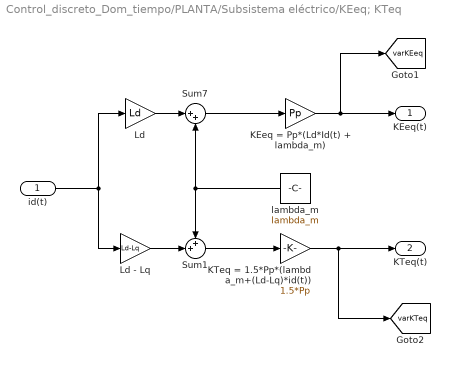
== system Control_discreto_Dom_tiempo/PLANTA/Subsistema eléctrico/KEeq; KTeq ==
  id(t) : Inport
  "KEeq = Pp*(Ld*Id(t) + lambda_m) " : Gain  Gain=Pp
  "KTeq = 1.5*Pp*(lambda_m+(Ld-Lq)*id(t)) " : Gain  Gain=1.5*Pp
  Ld : Gain  Gain=Ld
  Ld - Lq : Gain  Gain=Ld-Lq
  Sum1 : Sum  Inputs=++|
  Sum7 : Sum  Inputs=|++
  lambda_m : Constant  Value=lambda_m
  KEeq(t) : Outport
  KTeq(t) : Outport  Port=2
  tag scope: varKEeq=global, varKTeq=global
  wires:
  Ld/1 -> Sum7/1
  Sum7/1 -> "KEeq = Pp*(Ld*Id(t) + lambda_m) "/1
  "KTeq = 1.5*Pp*(lambda_m+(Ld-Lq)*id(t)) "/1 -> KTeq(t)/1, [varKTeq]
  Sum1/1 -> "KTeq = 1.5*Pp*(lambda_m+(Ld-Lq)*id(t)) "/1
  id(t)/1 -> Ld/1, Ld - Lq/1
  Ld - Lq/1 -> Sum1/2
  lambda_m/1 -> Sum1/1, Sum7/2
  "KEeq = Pp*(Ld*Id(t) + lambda_m) "/1 -> [varKEeq], KEeq(t)/1

== system Control_discreto_Dom_tiempo/PLANTA/Subsistema eléctrico/Park Transform1 ==
  abc : Inport
  theta : Inport  Port=2
  0 : Fcn  Expr=K1*(u(1) + u(2) + u(3))
  Gain1 : Gain  Gain=K2
  Mux2 : Mux  Inputs=2
  Mux3 : Mux  Inputs=3
  d : Fcn  Expr=sin(u(4)+Offset)*u(1) + sin(u(4)+Offset-2*pi/3)*u(2) + sin(u(4)+Offset+2*pi/3)*u(3)
  q : Fcn  Expr=cos(u(4)+Offset)*u(1) + cos(u(4)+Offset-2*pi/3)*u(2) + cos(u(4)+Offset+2*pi/3)*u(3)
  dq0 : Outport  VectorParamsAs1DForOutWhenUnconnected=off
  wires:
  0/1 -> Mux3/3
  Gain1/1 -> dq0/1
  Mux3/1 -> Gain1/1
  Mux2/1 -> 0/1, q/1, d/1
  theta/1 -> Mux2/2
  q/1 -> Mux3/2
  d/1 -> Mux3/1
  abc/1 -> Mux2/1
